simulink model "mdl01_antiwindup"  (R2021a)
settings: Solver=FixedStepAuto  StartTime=0.0  StopTime=10.0  FixedStep=Ts  RelTol=1e-3
values from neighbouring files (symbols this model uses):
  intLim = 3    [Sim01_antiwindup.m]    (also in Sim02_ctrlCompare.m = 1)
  Ka = 500    [Sim01_antiwindup.m]    (also in Sim02_ctrlCompare.m = 50)
  stepAmp = [1, -1]    [Sim01_antiwindup.m]    (also in Sim02_ctrlCompare.m = [0 1])
  stepTime = 5    [Sim01_antiwindup.m]    (also in Sim02_ctrlCompare.m = 0)
settings Model: Creator=xiaocy  LastModifiedBy=xiaocy
settings DataIOCC: ReturnWorkspaceOutputs=off

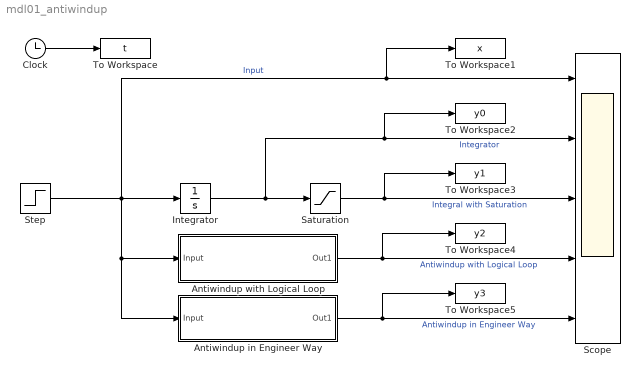
== system mdl01_antiwindup ==
  Antiwindup in Engineer Way : Subsystem
      mask Display: disp('Antiwindup Integrator\n(Engineer Way)')
  Antiwindup with Logical Loop : Subsystem
      mask Display: disp('Antiwindup Integrator\n(Logical)')
  Clock : Clock
  Integrator : Integrator
  Saturation : Saturate  UpperLimit=intLim  LowerLimit=-intLim
  Scope : Scope  NumInputPorts=5
  Step : Step  Time=stepTime  Before=stepAmp(1)  After=stepAmp(2)  SampleTime=0
  To Workspace : ToWorkspace  VariableName=t  SampleTime=-1
  To Workspace1 : ToWorkspace  VariableName=x  SampleTime=-1
  To Workspace2 : ToWorkspace  VariableName=y0  SampleTime=-1
  To Workspace3 : ToWorkspace  VariableName=y1  SampleTime=-1
  To Workspace4 : ToWorkspace  VariableName=y2  SampleTime=-1
  To Workspace5 : ToWorkspace  VariableName=y3  SampleTime=-1
  wires:
  Step/1 -> To Workspace1/1, Scope/1, Antiwindup in Engineer Way/1(Input), Antiwindup with Logical Loop/1(Input), Integrator/1  "Input"
  Integrator/1 -> To Workspace2/1, Scope/2, Saturation/1  "Integrator"
  Saturation/1 -> To Workspace3/1, Scope/3  "Integral with Saturation"
  Antiwindup with Logical Loop/1(Out1) -> To Workspace4/1, Scope/4  "Antiwindup with Logical Loop"
  Antiwindup in Engineer Way/1(Out1) -> To Workspace5/1, Scope/5  "Antiwindup in Engineer Way"
  Clock/1 -> To Workspace/1

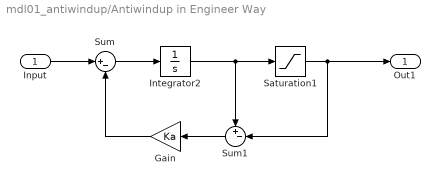
== system mdl01_antiwindup/Antiwindup in Engineer Way ==
  Input : Inport
  Gain : Gain  Gain=Ka
  Integrator2 : Integrator
  Saturation1 : Saturate  UpperLimit=intLim  LowerLimit=-intLim
  Sum : Sum  Inputs=|+-
  Sum1 : Sum  Inputs=+-|
  Out1 : Outport
  wires:
  Gain/1 -> Sum/2
  Sum1/1 -> Gain/1
  Integrator2/1 -> Saturation1/1, Sum1/1
  Sum/1 -> Integrator2/1
  Saturation1/1 -> Out1/1, Sum1/2
  Input/1 -> Sum/1

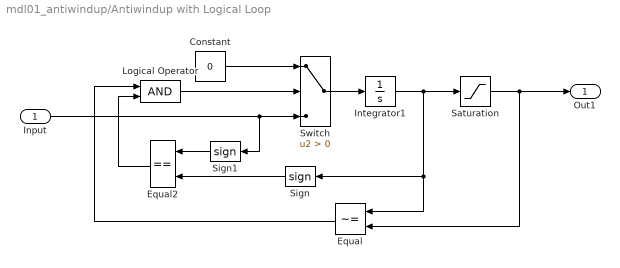
== system mdl01_antiwindup/Antiwindup with Logical Loop ==
  Input : Inport
  Constant : Constant  Value=0
  Equal : RelationalOperator  Operator=~=  OutDataTypeStr=boolean  RndMeth=Simplest
  Equal2 : RelationalOperator  Operator===  OutDataTypeStr=boolean  RndMeth=Simplest
  Integrator1 : Integrator  UpperSaturationLimit=intLim  LowerSaturationLimit=-intLim
  Logical Operator : Logic  AllPortsSameDT=off  OutDataTypeStr=boolean
  Saturation : Saturate  UpperLimit=intLim  LowerLimit=-intLim
  Sign : Signum
  Sign1 : Signum
  Switch : Switch  Criteria=u2 > Threshold
  Out1 : Outport
  wires:
  Integrator1/1 -> Saturation/1, Equal/1, Sign/1
  Saturation/1 -> Out1/1, Equal/2
  Input/1 -> Sign1/1, Switch/3
  Switch/1 -> Integrator1/1
  Sign/1 -> Equal2/2
  Sign1/1 -> Equal2/1
  Logical Operator/1 -> Switch/2
  Constant/1 -> Switch/1
  Equal/1 -> Logical Operator/1
  Equal2/1 -> Logical Operator/2
